simulink model "system"  (R2023a)
settings: Solver=ode15s  StartTime=0.0  StopTime=10.0  MaxStep=1e-3  RelTol=1e-3
libraries: fl_lib x6, nesl_utility x3, slpidlib x1, simulink x1
settings Model: Creator=LENOVO  LastModifiedBy=delto
settings DataIOCC: SaveOutput=off  SignalLogging=off  DSMLogging=off  ReturnWorkspaceOutputs=off  TimeSaveName=t
settings DebuggingCC: AlgebraicLoopMsg=none  ArtificialAlgebraicLoopMsg=none  OperatingPointInterfaceChecksumMismatchMsg=none

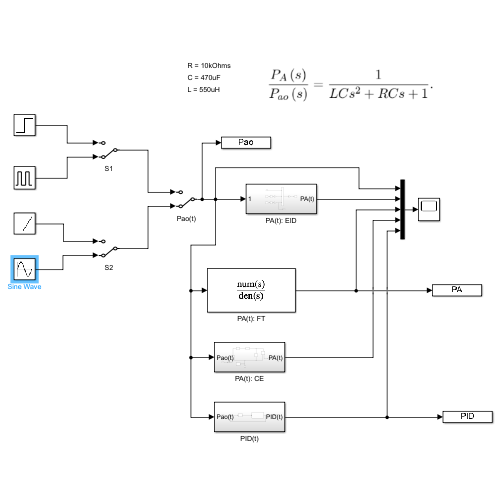
[thumbnail: Simulink's stored preview of the top-level diagram]
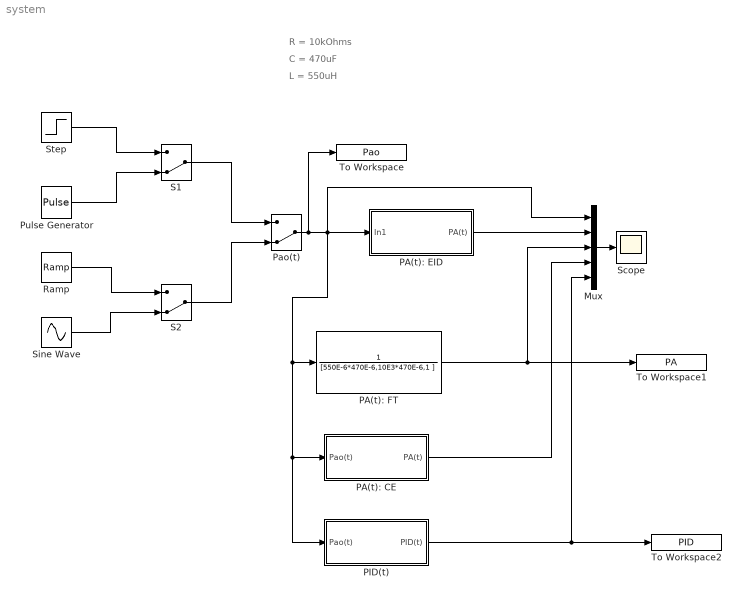
== system system ==
  note: L = 550uH
  note: C = 470uF
  note: R = 10kOhms
  Mux : Mux  Inputs=5
  PA(t): CE : Subsystem
  PA(t): EID : Subsystem
  PA(t): FT : TransferFcn  Denominator=[550E-6*470E-6,10E3*470E-6,1 ]
  PID(t) : Subsystem
  Pao(t) : ManualSwitch  CurrentSetting=0
  Pulse Generator : DiscretePulseGenerator  PulseType=Time based  Period=10  PulseWidth=10  PhaseDelay=1
  Ramp : simulink/Sources/Ramp  slope=1/10  start=0  InitialOutput=0
  S1 : ManualSwitch  CurrentSetting=0
  S2 : ManualSwitch  CurrentSetting=0
  Scope : Scope
  Sine Wave : Sin  Frequency=pi/2
  Step : Step  Time=0  SampleTime=0
  To Workspace : ToWorkspace  VariableName=Pao  SampleTime=-1
  To Workspace1 : ToWorkspace  VariableName=PA  SampleTime=-1
  To Workspace2 : ToWorkspace  VariableName=PID  SampleTime=-1
  wires:
  PA(t): EID/1(PA(t)) -> Mux/2
  Mux/1 -> Scope/1
  Step/1 -> S1/1
  Pao(t)/1 -> To Workspace/1, Mux/1, PID(t)/1(Pao(t)), PA(t): CE/1(Pao(t)), PA(t): FT/1, PA(t): EID/1(In1)
  S1/1 -> Pao(t)/1
  Pulse Generator/1 -> S1/2
  S2/1 -> Pao(t)/2
  Ramp/1 -> S2/1
  Sine Wave/1 -> S2/2
  PA(t): FT/1 -> Mux/3, To Workspace1/1
  PA(t): CE/1(PA(t)) -> Mux/4
  PID(t)/1(PID(t)) -> To Workspace2/1, Mux/5

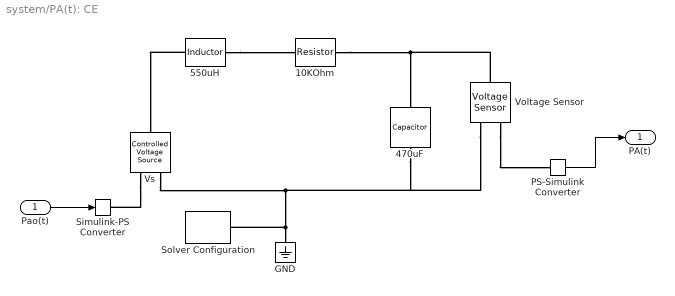
== system system/PA(t): CE ==
  Pao(t) : Inport
  10KOhm : fl_lib/Electrical/Electrical Elements/Resistor  R=10 kOhm  i_specify=off  i_priority=None  i=0 A  i_nominal_specify=off  i_nominal_unit=A  i_nominal_value=1  v_specify=off  v_priority=None  v=0 V  v_nominal_specify=off  v_nominal_unit=V  v_nominal_value=1
  470uF : fl_lib/Electrical/Electrical Elements/Capacitor  c=470e-6 F  r=1e-6 Ohm  g=0 1/Ohm  i_specify=off  i_priority=None  i=0 A  i_nominal_specify=off  i_nominal_unit=A  i_nominal_value=1  v_specify=off  v_priority=None  v=0 V  v_nominal_specify=off  v_nominal_unit=V  v_nominal_value=1  vc_specify=off  vc_priority=High  vc=0 V  vc_nominal_specify=off  vc_nominal_unit=V  vc_nominal_value=1
  550uH : fl_lib/Electrical/Electrical Elements/Inductor  l=550e-6 H  r=0 Ohm  g=1e-9 1/Ohm  i_specify=off  i_priority=None  i=0 A  i_nominal_specify=off  i_nominal_unit=A  i_nominal_value=1  v_specify=off  v_priority=None  v=0 V  v_nominal_specify=off  v_nominal_unit=V  v_nominal_value=1  i_L_specify=off  i_L_priority=High  i_L=0 A  i_L_nominal_specify=off  i_L_nominal_unit=A  i_L_nominal_value=1
  GND : fl_lib/Electrical/Electrical Elements/Electrical Reference
  PS-Simulink Converter : nesl_utility/PS-Simulink Converter  PhysicalDomain=network_engine_domain  SubClassName=ps_output  LeftPortType=input  RightPortType=output  PseudoPeriodic=off  Frequencies=[]  VectorFormat=inherit  Unit=inherit  AffineConversion=off
  Simulink-PS Converter : nesl_utility/Simulink-PS Converter  PhysicalDomain=network_engine_domain  SubClassName=ps_input  LeftPortType=input  RightPortType=output  PseudoPeriodic=off  Frequencies=[]  NoiseDistribution=none  NoiseParameters=[]  Unit=1  AffineConversion=off  FilteringAndDerivatives=provide  SimscapeFilterOrder=1  InputFilterTimeConstant=0.001  UdotUserProvided=0
  Solver Configuration : nesl_utility/Solver Configuration  PhysicalDomain=network_engine_domain  SubClassName=solver  LeftPortType=input  RightPortType=generic  Tones=[]  Harmonics=[]  SimulateNoise=off  Profile=off  UseLocalSampling=off  EnableSwitchedLinearOptims=on  FrequencyDomain=off  UseCCode=off  RelTol=0.001  AbsTol=0.001  MinStep=1e-09  ToWorkspace=off  RevertToSquareIcSolve=off  NumHomotopyIterations=100  PhasorMode=off  PhasorModeNumHarmonics=1  ConsistencySolver=NEWTON_XTOL_AFTER_FTOL  IndexReductionMethod=DerivativeReplacement  DoDC=off  ResidualTolerance=1e-09  ConsistencyTolSource=GLOBAL  ConsistencyAbsTol=0.001  ConsistencyRelTol=0.001  ConsistencyTolFactor=0.001  UseLocalSolver=off  LocalSolverChoice=NE_BACKWARD_EULER_ADVANCER  ResolveIndetEquations=on  FunctionEvalNumThread=1  LocalSolverSampleTime=0.001  DoFixedCost=off  MaxNonlinIter=3  MaxModeIter=2  ComputeImpulses=off  ImpulseIterations=2  LinearAlgebra=auto  LinearAlgebraNumThread=0  EquationFormulation=NE_TIME_EF  DelaysMemoryBudget=1024  AutomaticFiltering=on  FilteringTimeConstant=0.001  PartitionStorageMethod=AS_NEEDED  PartitionMemoryBudget=1024  PartitionMethod=ROBUST
  Voltage Sensor : fl_lib/Electrical/Electrical Sensors/Voltage Sensor
  Vs : fl_lib/Electrical/Electrical Sources/Controlled Voltage Source
  PA(t) : Outport
  wires:
  Pao(t)/1 -> Simulink-PS Converter/1
  PS-Simulink Converter/1 -> PA(t)/1
  connections:
  Vs/RConn1 -- Simulink-PS Converter/RConn1
  550uH/LConn1 -- Vs/LConn1
  550uH/RConn1 -- 10KOhm/LConn1
  10KOhm/RConn1 -- Voltage Sensor/LConn1 -- 470uF/LConn1
  Vs/RConn2 -- Voltage Sensor/RConn2 -- 470uF/RConn1 -- Solver Configuration/RConn1 -- GND/LConn1
  Voltage Sensor/RConn1 -- PS-Simulink Converter/LConn1

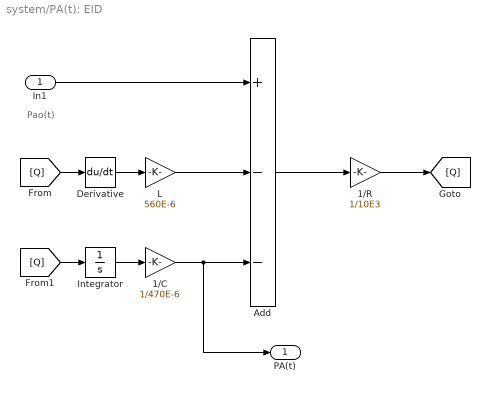
== system system/PA(t): EID ==
  note: Pao(t)
  In1 : Inport
  1/C : Gain  Gain=1/470E-6
  1/R : Gain  Gain=1/10E3
  Add : Sum  Inputs=+--
  Derivative : Derivative
  Integrator : Integrator
  L : Gain  Gain=560E-6
  PA(t) : Outport
  wires:
  In1/1 -> Add/1
  Derivative/1 -> L/1
  L/1 -> Add/2
  Integrator/1 -> 1/C/1
  1/C/1 -> PA(t)/1, Add/3
  Add/1 -> 1/R/1
  [Q] -> Derivative/1
  [Q] -> Integrator/1
  1/R/1 -> [Q]

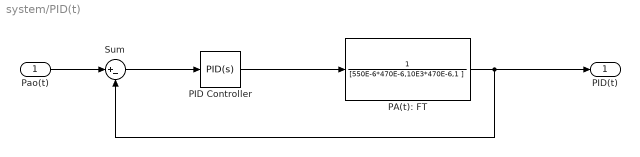
== system system/PID(t) ==
  Pao(t) : Inport
  PA(t): FT : TransferFcn  Denominator=[550E-6*470E-6,10E3*470E-6,1 ]
  PID Controller : slpidlib/PID Controller  Controller=PID  Form=Parallel  TimeDomain=Continuous-time  UseExternalTs=off  SampleTime=-1  IntegratorMethod=Forward Euler  FilterMethod=Forward Euler  ControllerParametersSource=internal  P=564.07358955857  I=13492.8531425784  UseKiTs=off  D=-1.24837012884727  N=451.84803490887  UseFilter=on  TunerSelectOption=Transfer Function Based (PID Tuner App)  InitialConditionSource=internal  InitialConditionForIntegrator=0  InitialConditionForFilter=0  DifferentiatorICPrevScaledInput=0  ExternalReset=none  TrackingMode=off  Kt=1  LimitOutput=off  SatLimitsSource=internal  UpperSaturationLimit=inf  LowerSaturationLimit=-inf  LinearizeAsGain=on  AntiWindupMode=none  Kb=1  LimitIntegrator=off  UpperIntegratorSaturationLimit=inf  LowerIntegratorSaturationLimit=-inf  POutMin=[]  POutMax=[]  IOutMin=[]  IOutMax=[]  DOutMin=[]  DOutMax=[]  NOutMin=[]  NOutMax=[]  SumOutMin=[]  SumOutMax=[]  SaturationOutMin=[]  SaturationOutMax=[]  PParamMin=[]  PParamMax=[]  IParamMin=[]  IParamMax=[]  DParamMin=[]  DParamMax=[]  NParamMin=[]  NParamMax=[]  KbParamMin=[]  KbParamMax=[]  KtParamMin=[]  KtParamMax=[]  KbOutMin=[]  KbOutMax=[]  KtOutMin=[]  KtOutMax=[]  IntegratorOutMin=[]  IntegratorOutMax=[]  FilterOutMin=[]  FilterOutMax=[]  SumI1OutMin=[]  SumI1OutMax=[]  SumI2OutMin=[]  SumI2OutMax=[]  SumI3OutMin=[]  SumI3OutMax=[]  SumI4OutMin=[]  SumI4OutMax=[]  SumDOutMin=[]  SumDOutMax=[]  DifferentiatorOutMin=[]  DifferentiatorOutMax=[]  FilterDiffOutCoefMin=[]  FilterDiffOutCoefMax=[]  ReciprocalOutMin=[]  ReciprocalOutMax=[]  SumDenOutMin=[]  SumDenOutMax=[]  SumNumOutMin=[]  SumNumOutMax=[]  DivideOutMin=[]  DivideOutMax=[]  UdiffTsProdOutMin=[]  UdiffTsProdOutMax=[]  NTsProdOutMin=[]  NTsProdOutMax=[]  UintegralTsProdOutMin=[]  UintegralTsProdOutMax=[]  UngainTsProdOutMin=[]  UngainTsProdOutMax=[]  ClampingZeroOutDataTypeStr=Inherit: Inherit via back propagation  ClampingZeroOutMin=[]  ClampingZeroOutMax=[]  FilterDenConstantOutDataTypeStr=Inherit: Inherit via back propagation  FilterDenConstantOutMin=[]  FilterDenConstantOutMax=[]  PCopyOutDataTypeStr=Inherit: Inherit via back propagation  PCopyOutMin=[]  PCopyOutMax=[]  NCopyOutDataTypeStr=Inherit: Inherit via back propagation  NCopyOutMin=[]  NCopyOutMax=[]  IntegratorContinuousStateAttributes=''  IntegratorStateMustResolveToSignalObject=off  IntegratorRTWStateStorageClass=Auto  FilterContinuousStateAttributes=''  FilterStateMustResolveToSignalObject=off  FilterRTWStateStorageClass=Auto  ParallelPVariant=InternalParameters  IdealPVariant=Disabled  IVariant=InternalParameters  DVariant=InternalParameters  IntegratorVariant=Continuous  SatVariant=Disabled  AWVariant=Passthrough  PCopyVariant=Disabled  TRVariant=Disabled  FdbkBlocksVariant=Forward  IdealPFdbkVariant=Disabled  SatFdbkVariant=Disabled  DerivativeFilterVariant=ContFilter  NVariant=InternalParameters  NCopyVariant=Disabled  FilterICVariant=InternalICsFilter  IntegratorICVariant=InternalICs  ExternalResetVariant=Disabled  TRSumVariant=Passthrough  SumFdbkVariant=Disabled  SumVariant=Sum_PID  TsampFilterVariant=InternalTs  TsampNgainVariant=Passthrough  TsampIntegralVariant=Disabled_SignalSpec  ExternalSaturationOutDataTypeStr=Inherit: Same as second input
  Sum : Sum  Inputs=|+-
  PID(t) : Outport
  wires:
  PA(t): FT/1 -> PID(t)/1, Sum/2
  PID Controller/1 -> PA(t): FT/1
  Sum/1 -> PID Controller/1
  Pao(t)/1 -> Sum/1
